simulink model "underwater"  (Simulink 5.1)
settings: Solver=ode45  StartTime=0.0  StopTime=10.0  RelTol=1e-3
settings Model: LastModifiedBy=beard  BooleanDataType=on  ProdHWDeviceType=Microprocessor

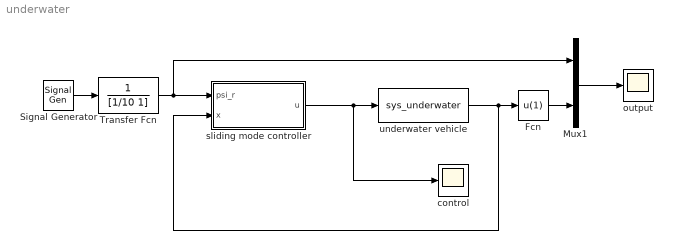
== system underwater ==
  Fcn : Fcn  Expr=u(1)
  Mux1 : Mux  Inputs=2
  Signal Generator : SignalGenerator  WaveForm=square  Frequency=.1
  Transfer Fcn : TransferFcn  Denominator=[1/10 1]
  control : Scope
      settings: YMin=-25  YMax=50
  output : Scope
      settings: YMin=-1.1  YMax=1
  sliding mode controller : Subsystem
  underwater vehicle : S-Function  FunctionName=sys_underwater
  wires:
  underwater vehicle/1 -> sliding mode controller/2(x), Fcn/1
  Signal Generator/1 -> Transfer Fcn/1
  Mux1/1 -> output/1
  sliding mode controller/1(u) -> underwater vehicle/1, control/1
  Fcn/1 -> Mux1/2
  Transfer Fcn/1 -> Mux1/1, sliding mode controller/1(psi_r)

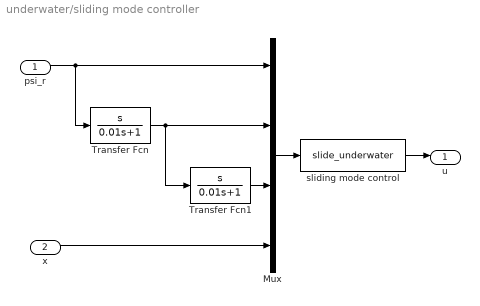
== system underwater/sliding mode controller ==
  psi_r : Inport
  x : Inport  Port=2
  Mux : Mux
  Transfer Fcn : TransferFcn  Numerator=[1 0]  Denominator=[0.01 1]
  Transfer Fcn1 : TransferFcn  Numerator=[1 0]  Denominator=[0.01 1]
  sliding mode control : S-Function  FunctionName=slide_underwater
  u : Outport
  wires:
  Mux/1 -> sliding mode control/1
  psi_r/1 -> Mux/1, Transfer Fcn/1
  sliding mode control/1 -> u/1
  x/1 -> Mux/4
  Transfer Fcn/1 -> Mux/2, Transfer Fcn1/1
  Transfer Fcn1/1 -> Mux/3
